simulink model "RS_O_yalmip"  (R2016b)
settings: Solver=ode1  StartTime=0.0  StopTime=T  FixedStep=1e-4  MaxStep=1e-3  RelTol=1e-6  EnableMultiTasking=on
InitFcn:
  | RS_O_script;
values from neighbouring files (symbols this model uses):
  C1 = 1e-9    (= 1e-09)    [Dati_MPC.m]
  C2 = 1e-9    (= 1e-09)    [Dati_MPC.m]
  Cext_Bp1 = Ce_Bp1*np_Bp1/ns_Bp1    (= 35750)    [Dati_MPC.m]
  Cext_Bp2 = Ce_Bp2*np_Bp2/ns_Bp2    (= 35750)    [Dati_MPC.m]
  Cext_BpM = Ce_BpM*np_BpM/ns_BpM    (= 68250)    [Dati_MPC.m]
  Cin_Bp1 = Ci_Bp1*np_Bp1/ns_Bp1    (= 16500)    [Dati_MPC.m]
  Cin_Bp2 = Ci_Bp2*np_Bp2/ns_Bp2    (= 16500)    [Dati_MPC.m]
  Cin_BpM = Ci_BpM*np_BpM/ns_BpM    (= 31500)    [Dati_MPC.m]
  Cint = 18e-3    (= 0.018)    [Dati_MPC.m]
  f = 50    [Dati_rete.m]
  ft_F = 10    [Dati_MPC.m]
  I_u = 0.1    [Dati_MPC.m]
  ki_PLL = w_t/Vd*(-w_t+sqrt(2*w_t^2-Vd^2*kp_PLL^2))    [Dati_MPC.m]
  kp_PLL = 0.9*kp_PLL_max    [Dati_MPC.m]
  MPCpar = struct    [Dati_MPC.m]    (also in Initialization.m)
  netdata = struct    [Dati_rete.m]
  P1 = 750e3    (= 750000)    [RS_O_script.m]
  P1v = 500e3    (= 500000)    [RS_O_script.m]
  P2 = 750e3    (= 750000)    [RS_O_script.m]
  P2v = 250e3    (= 250000)    [RS_O_script.m]
  P_u = 0.005    [Dati_MPC.m]
  Ppv1 = 500e3    (= 500000)    [Dati_MPC.m]
  Ppv2 = 850e3    (= 850000)    [Dati_MPC.m]
  Q1 = 350e3    (= 350000)    [RS_O_script.m]
  Q1v = 250e3    (= 250000)    [RS_O_script.m]
  Q2 = 300e3    (= 300000)    [RS_O_script.m]
  Q2v = 250e3    (= 250000)    [RS_O_script.m]
  Qbat1 = 50e3    (= 50000)    [Dati_MPC.m]
  Qbat2 = 50e3    (= 50000)    [Dati_MPC.m]
  Rext_Bp1 = Re_Bp1*ns_Bp1/np_Bp1    (= 0.0154545454545)    [Dati_MPC.m]
  Rext_Bp2 = Re_Bp2*ns_Bp2/np_Bp2    (= 0.0154545454545)    [Dati_MPC.m]
  Rext_BpM = Re_BpM*ns_BpM/np_BpM    (= 0.00809523809524)    [Dati_MPC.m]
  Rin_Bp1 = Ri_Bp1*ns_Bp1/np_Bp1    (= 0.363636363636)    [Dati_MPC.m]
  Rin_Bp2 = Ri_Bp2*ns_Bp2/np_Bp2    (= 0.363636363636)    [Dati_MPC.m]
  Rin_BpM = Ri_BpM*ns_BpM/np_BpM    (= 0.190476190476)    [Dati_MPC.m]
  SOC_10 = (Vbat1-Vbat1_min)/(Vbat1_max-Vbat1_min)    (= 0.625)    [Dati_MPC.m]
  SOC_20 = (Vbat2-Vbat2_min)/(Vbat2_max-Vbat2_min)    (= 0.625)    [Dati_MPC.m]
  SOC_M0 = (VbatM-VbatM_min)/(VbatM_max-VbatM_min)    (= 0.625)    [Dati_MPC.m]
  Srif = 1e6    (= 1000000)    [Dati_rete.m]
  t1 = 50    [RS_O_script.m]
  t2 = 110    [RS_O_script.m]
  t3 = 170    [RS_O_script.m]
  t_start_MPC = 10    [RS_O_script.m]
  tPLL = 2    [RS_O_script.m]
  Vbat1_max = 1.2*Vbat1_min    (= 480)    [Dati_MPC.m]
  Vbat1_min = 400    [Dati_MPC.m]
  Vbat2_max = 1.2*Vbat2_min    (= 480)    [Dati_MPC.m]
  Vbat2_min = 400    [Dati_MPC.m]
  VbatM_max = 1.2*VbatM_min    (= 480)    [Dati_MPC.m]
  VbatM_min = 400    [Dati_MPC.m]
  Vdc_1 = 800    [Dati_MPC.m]
  Vdc_2 = 800    [Dati_MPC.m]
  Vdc_M = 800    [Dati_MPC.m]
  Vrif_M = sqrt(2)/sqrt(3)*20e3    [Dati_MPC.m]
  Zrif = Vrif^2/Srif    (= 400)    [Dati_rete.m]
undefined symbols (not defined in the file or in its folder): Cfsc, Csc, j, L2, Lf, magnitude, Rc, Rint, Rsc
libraries: powerlib x87, powerlib_meascontrol x58, simulink x2
(part 3 of 3)

== system RS_O_yalmip/Misure 1/Filtro_c ==
  In : Inport
  Complex to Real-Imag : ComplexToRealImag
  First-Order Filter : powerlib_meascontrol/Filters/First-Order Filter  FilterType=Lowpass  Tc=1/(2*pi*ft_F)  Ts=0  Initialize=on  Vac_Init=[0, 0, 60]  Vdc_Init=0  PlotResponse=off  FreqRange="[0,  200,  1]"
  First-Order Filter1 : powerlib_meascontrol/Filters/First-Order Filter  FilterType=Lowpass  Tc=1/(2*pi*ft_F)  Ts=0  Initialize=on  Vac_Init=[0, 0, 60]  Vdc_Init=0  PlotResponse=off  FreqRange="[0,  200,  1]"
  Real-Imag to Complex : RealImagToComplex
  Out : Outport
  wires:
  Complex to Real-Imag/2 -> First-Order Filter1/1
  First-Order Filter/1 -> Real-Imag to Complex/1
  Complex to Real-Imag/1 -> First-Order Filter/1
  First-Order Filter1/1 -> Real-Imag to Complex/2
  Real-Imag to Complex/1 -> Out/1
  In/1 -> Complex to Real-Imag/1

== system RS_O_yalmip/Misure 1/Filtro_c1 ==
  In : Inport
  Complex to Real-Imag : ComplexToRealImag
  First-Order Filter : powerlib_meascontrol/Filters/First-Order Filter  FilterType=Lowpass  Tc=1/(2*pi*ft_F)  Ts=0  Initialize=on  Vac_Init=[0, 0, 60]  Vdc_Init=0  PlotResponse=off  FreqRange="[0,  200,  1]"
  First-Order Filter1 : powerlib_meascontrol/Filters/First-Order Filter  FilterType=Lowpass  Tc=1/(2*pi*ft_F)  Ts=0  Initialize=on  Vac_Init=[0, 0, 60]  Vdc_Init=0  PlotResponse=off  FreqRange="[0,  200,  1]"
  Real-Imag to Complex : RealImagToComplex
  Out : Outport
  wires:
  In/1 -> Complex to Real-Imag/1
  Real-Imag to Complex/1 -> Out/1
  First-Order Filter1/1 -> Real-Imag to Complex/2
  Complex to Real-Imag/1 -> First-Order Filter/1
  First-Order Filter/1 -> Real-Imag to Complex/1
  Complex to Real-Imag/2 -> First-Order Filter1/1

== system RS_O_yalmip/Misure 1/I Park assi sincroni1 ==
  I_1,2,3 : Inport
  Fase_rete : Inport  Port=2
  Add : Sum  Inputs=+++
  Constant : Constant  Value=exp(j*2*pi/3)
  Constant1 : Constant  Value=exp(j*4*pi/3)
  Demux : Demux  Outputs=3
  Gain : Gain  Gain=2/3
  Gain1 : Gain  Gain=-j
  Math Function : Math  SaturateOnIntegerOverflow=on
  Product : Product
  Product1 : Product
  Product2 : Product
  I_d,q : Outport
  wires:
  Math Function/1 -> Product2/2
  Fase_rete/1 -> Gain1/1
  Product2/1 -> I_d,q/1
  Gain1/1 -> Math Function/1
  Gain/1 -> Product2/1
  Product/1 -> Add/2
  Product1/1 -> Add/3
  Constant/1 -> Product/2
  Constant1/1 -> Product1/2
  Add/1 -> Gain/1
  I_1,2,3/1 -> Demux/1
  Demux/1 -> Add/1
  Demux/2 -> Product/1
  Demux/3 -> Product1/1

== system RS_O_yalmip/Misure 1/Subsystem1 ==
  V_dq : Inport
  I_dq : Inport  Port=2
  Divide2 : Product  Inputs=**
  Gain : Gain  Gain=3/2
  Math Function : Math  Operator=conj  SaturateOnIntegerOverflow=on
  P,Q : Outport
  wires:
  Divide2/1 -> Gain/1
  Gain/1 -> P,Q/1
  Math Function/1 -> Divide2/2
  V_dq/1 -> Divide2/1
  I_dq/1 -> Math Function/1

== system RS_O_yalmip/Misure 1/V Park assi sincroni ==
  V_c_1,2,3 : Inport
  Fase_rete : Inport  Port=2
  Add : Sum  Inputs=+++
  Constant : Constant  Value=exp(j*2*pi/3)
  Constant1 : Constant  Value=exp(j*4*pi/3)
  Demux : Demux  Outputs=3
  Gain : Gain  Gain=2/3
  Gain1 : Gain  Gain=-j
  Math Function : Math  SaturateOnIntegerOverflow=on
  Product : Product
  Product1 : Product
  Product2 : Product
  Vc_d,q : Outport
  wires:
  Gain/1 -> Product2/1
  Demux/3 -> Product1/1
  Demux/2 -> Product/1
  Demux/1 -> Add/1
  V_c_1,2,3/1 -> Demux/1
  Add/1 -> Gain/1
  Constant1/1 -> Product1/2
  Constant/1 -> Product/2
  Product1/1 -> Add/3
  Product/1 -> Add/2
  Math Function/1 -> Product2/2
  Gain1/1 -> Math Function/1
  Product2/1 -> Vc_d,q/1
  Fase_rete/1 -> Gain1/1

== system RS_O_yalmip/Misure 2/Filtro_c ==
  In : Inport
  Complex to Real-Imag : ComplexToRealImag
  First-Order Filter : powerlib_meascontrol/Filters/First-Order Filter  FilterType=Lowpass  Tc=1/(2*pi*ft_F)  Ts=0  Initialize=on  Vac_Init=[0, 0, 60]  Vdc_Init=0  PlotResponse=off  FreqRange="[0,  200,  1]"
  First-Order Filter1 : powerlib_meascontrol/Filters/First-Order Filter  FilterType=Lowpass  Tc=1/(2*pi*ft_F)  Ts=0  Initialize=on  Vac_Init=[0, 0, 60]  Vdc_Init=0  PlotResponse=off  FreqRange="[0,  200,  1]"
  Real-Imag to Complex : RealImagToComplex
  Out : Outport
  wires:
  Complex to Real-Imag/2 -> First-Order Filter1/1
  First-Order Filter/1 -> Real-Imag to Complex/1
  Complex to Real-Imag/1 -> First-Order Filter/1
  First-Order Filter1/1 -> Real-Imag to Complex/2
  Real-Imag to Complex/1 -> Out/1
  In/1 -> Complex to Real-Imag/1

== system RS_O_yalmip/Misure 2/Filtro_c1 ==
  In : Inport
  Complex to Real-Imag : ComplexToRealImag
  First-Order Filter : powerlib_meascontrol/Filters/First-Order Filter  FilterType=Lowpass  Tc=1/(2*pi*ft_F)  Ts=0  Initialize=on  Vac_Init=[0, 0, 60]  Vdc_Init=0  PlotResponse=off  FreqRange="[0,  200,  1]"
  First-Order Filter1 : powerlib_meascontrol/Filters/First-Order Filter  FilterType=Lowpass  Tc=1/(2*pi*ft_F)  Ts=0  Initialize=on  Vac_Init=[0, 0, 60]  Vdc_Init=0  PlotResponse=off  FreqRange="[0,  200,  1]"
  Real-Imag to Complex : RealImagToComplex
  Out : Outport
  wires:
  In/1 -> Complex to Real-Imag/1
  Real-Imag to Complex/1 -> Out/1
  First-Order Filter1/1 -> Real-Imag to Complex/2
  Complex to Real-Imag/1 -> First-Order Filter/1
  First-Order Filter/1 -> Real-Imag to Complex/1
  Complex to Real-Imag/2 -> First-Order Filter1/1

== system RS_O_yalmip/Misure 2/I Park assi sincroni1 ==
  I_1,2,3 : Inport
  Fase_rete : Inport  Port=2
  Add : Sum  Inputs=+++
  Constant : Constant  Value=exp(j*2*pi/3)
  Constant1 : Constant  Value=exp(j*4*pi/3)
  Demux : Demux  Outputs=3
  Gain : Gain  Gain=2/3
  Gain1 : Gain  Gain=-j
  Math Function : Math  SaturateOnIntegerOverflow=on
  Product : Product
  Product1 : Product
  Product2 : Product
  I_d,q : Outport
  wires:
  Demux/3 -> Product1/1
  Demux/2 -> Product/1
  Demux/1 -> Add/1
  I_1,2,3/1 -> Demux/1
  Add/1 -> Gain/1
  Constant1/1 -> Product1/2
  Constant/1 -> Product/2
  Product1/1 -> Add/3
  Product/1 -> Add/2
  Gain/1 -> Product2/1
  Gain1/1 -> Math Function/1
  Product2/1 -> I_d,q/1
  Fase_rete/1 -> Gain1/1
  Math Function/1 -> Product2/2

== system RS_O_yalmip/Misure 2/Subsystem1 ==
  V_dq : Inport
  I_dq : Inport  Port=2
  Divide2 : Product  Inputs=**
  Gain : Gain  Gain=3/2
  Math Function : Math  Operator=conj  SaturateOnIntegerOverflow=on
  P,Q : Outport
  wires:
  I_dq/1 -> Math Function/1
  V_dq/1 -> Divide2/1
  Math Function/1 -> Divide2/2
  Gain/1 -> P,Q/1
  Divide2/1 -> Gain/1

== system RS_O_yalmip/Misure 2/V Park assi sincroni ==
  V_c_1,2,3 : Inport
  Fase_rete : Inport  Port=2
  Add : Sum  Inputs=+++
  Constant : Constant  Value=exp(j*2*pi/3)
  Constant1 : Constant  Value=exp(j*4*pi/3)
  Demux : Demux  Outputs=3
  Gain : Gain  Gain=2/3
  Gain1 : Gain  Gain=-j
  Math Function : Math  SaturateOnIntegerOverflow=on
  Product : Product
  Product1 : Product
  Product2 : Product
  Vc_d,q : Outport
  wires:
  Fase_rete/1 -> Gain1/1
  Product2/1 -> Vc_d,q/1
  Gain1/1 -> Math Function/1
  Math Function/1 -> Product2/2
  Product/1 -> Add/2
  Product1/1 -> Add/3
  Constant/1 -> Product/2
  Constant1/1 -> Product1/2
  Add/1 -> Gain/1
  V_c_1,2,3/1 -> Demux/1
  Demux/1 -> Add/1
  Demux/2 -> Product/1
  Demux/3 -> Product1/1
  Gain/1 -> Product2/1

== system RS_O_yalmip/Misure Master/Filtro_c ==
  In : Inport
  Complex to Real-Imag : ComplexToRealImag
  First-Order Filter : powerlib_meascontrol/Filters/First-Order Filter  FilterType=Lowpass  Tc=1/(2*pi*ft_F)  Ts=0  Initialize=on  Vac_Init=[0, 0, 60]  Vdc_Init=0  PlotResponse=off  FreqRange="[0,  200,  1]"
  First-Order Filter1 : powerlib_meascontrol/Filters/First-Order Filter  FilterType=Lowpass  Tc=1/(2*pi*ft_F)  Ts=0  Initialize=on  Vac_Init=[0, 0, 60]  Vdc_Init=0  PlotResponse=off  FreqRange="[0,  200,  1]"
  Real-Imag to Complex : RealImagToComplex
  Out : Outport
  wires:
  Complex to Real-Imag/2 -> First-Order Filter1/1
  First-Order Filter/1 -> Real-Imag to Complex/1
  Complex to Real-Imag/1 -> First-Order Filter/1
  First-Order Filter1/1 -> Real-Imag to Complex/2
  Real-Imag to Complex/1 -> Out/1
  In/1 -> Complex to Real-Imag/1

== system RS_O_yalmip/Misure Master/Filtro_c1 ==
  In : Inport
  Complex to Real-Imag : ComplexToRealImag
  First-Order Filter : powerlib_meascontrol/Filters/First-Order Filter  FilterType=Lowpass  Tc=1/(2*pi*ft_F)  Ts=0  Initialize=on  Vac_Init=[0, 0, 60]  Vdc_Init=0  PlotResponse=off  FreqRange="[0,  200,  1]"
  First-Order Filter1 : powerlib_meascontrol/Filters/First-Order Filter  FilterType=Lowpass  Tc=1/(2*pi*ft_F)  Ts=0  Initialize=on  Vac_Init=[0, 0, 60]  Vdc_Init=0  PlotResponse=off  FreqRange="[0,  200,  1]"
  Real-Imag to Complex : RealImagToComplex
  Out : Outport
  wires:
  In/1 -> Complex to Real-Imag/1
  Real-Imag to Complex/1 -> Out/1
  First-Order Filter1/1 -> Real-Imag to Complex/2
  Complex to Real-Imag/1 -> First-Order Filter/1
  First-Order Filter/1 -> Real-Imag to Complex/1
  Complex to Real-Imag/2 -> First-Order Filter1/1

== system RS_O_yalmip/Misure Master/I Park assi sincroni1 ==
  I_1,2,3 : Inport
  Fase_rete : Inport  Port=2
  Add : Sum  Inputs=+++
  Constant : Constant  Value=exp(j*2*pi/3)
  Constant1 : Constant  Value=exp(j*4*pi/3)
  Demux : Demux  Outputs=3
  Gain : Gain  Gain=2/3
  Gain1 : Gain  Gain=-j
  Math Function : Math  SaturateOnIntegerOverflow=on
  Product : Product
  Product1 : Product
  Product2 : Product
  I_d,q : Outport
  I_ab : Outport  Port=2
  wires:
  Demux/3 -> Product1/1
  Demux/2 -> Product/1
  Demux/1 -> Add/1
  I_1,2,3/1 -> Demux/1
  Add/1 -> Gain/1
  Constant1/1 -> Product1/2
  Constant/1 -> Product/2
  Product1/1 -> Add/3
  Product/1 -> Add/2
  Gain/1 -> I_ab/1, Product2/1
  Gain1/1 -> Math Function/1
  Product2/1 -> I_d,q/1
  Fase_rete/1 -> Gain1/1
  Math Function/1 -> Product2/2

== system RS_O_yalmip/Misure Master/Subsystem1 ==
  V_dq : Inport
  I_dq : Inport  Port=2
  Divide2 : Product  Inputs=**
  Gain : Gain  Gain=3/2
  Math Function : Math  Operator=conj  SaturateOnIntegerOverflow=on
  P,Q : Outport
  wires:
  I_dq/1 -> Math Function/1
  V_dq/1 -> Divide2/1
  Math Function/1 -> Divide2/2
  Gain/1 -> P,Q/1
  Divide2/1 -> Gain/1

== system RS_O_yalmip/Misure Master/V Park assi sincroni ==
  V_c_1,2,3 : Inport
  Fase_rete : Inport  Port=2
  Add : Sum  Inputs=+++
  Constant : Constant  Value=exp(j*2*pi/3)
  Constant1 : Constant  Value=exp(j*4*pi/3)
  Demux : Demux  Outputs=3
  Gain : Gain  Gain=2/3
  Gain1 : Gain  Gain=-j
  Math Function : Math  SaturateOnIntegerOverflow=on
  Product : Product
  Product1 : Product
  Product2 : Product
  Vc_d,q : Outport
  wires:
  Fase_rete/1 -> Gain1/1
  Product2/1 -> Vc_d,q/1
  Gain1/1 -> Math Function/1
  Math Function/1 -> Product2/2
  Product/1 -> Add/2
  Product1/1 -> Add/3
  Constant/1 -> Product/2
  Constant1/1 -> Product1/2
  Add/1 -> Gain/1
  V_c_1,2,3/1 -> Demux/1
  Demux/1 -> Add/1
  Demux/2 -> Product/1
  Demux/3 -> Product1/1
  Gain/1 -> Product2/1

== system RS_O_yalmip/Misure transito/Subsystem2 ==
  V_c : Inport
  Add : Sum  Inputs=+-
  Add1 : Sum  Inputs=+-
  Add2 : Sum  Inputs=+-
  Demux : Demux  Outputs=3
  Gain : Gain  Gain=1/3
  Gain1 : Gain  Gain=1/3
  Gain2 : Gain  Gain=1/3
  Mux2 : Mux  Inputs=3
  V_f : Outport
  wires:
  Demux/3 -> Gain2/1
  V_c/1 -> Demux/1
  Add2/1 -> Mux2/3
  Add1/1 -> Mux2/2
  Add/1 -> Mux2/1
  Gain1/1 -> Add1/1, Add2/2
  Gain2/1 -> Add2/1, Add/2
  Demux/2 -> Gain1/1
  Gain/1 -> Add/1, Add1/2
  Demux/1 -> Gain/1
  Mux2/1 -> V_f/1

== system RS_O_yalmip/Carico1/PLL/Filtro_c ==
  In : Inport
  Complex to Real-Imag : ComplexToRealImag
  Real-Imag to Complex : RealImagToComplex
  Second-Order Filter{1..4} (4 alike) : powerlib_meascontrol/Filters/Second-Order Filter  FilterType=Lowpass  Fo=ft_PLL  Zeta=0.707  Ts=0  Initialize=on  Vac_Init="[0,  0,  60]"  Vdc_Init=Vrif_M  PlotResponse=off  FreqRange=[0, 500, 1]
  Out : Outport
  wires:
  Complex to Real-Imag/2 -> Second-Order Filter3/1
  Second-Order Filter3/1 -> Second-Order Filter4/1
  Second-Order Filter2/1 -> Real-Imag to Complex/1
  Second-Order Filter1/1 -> Second-Order Filter2/1
  Second-Order Filter4/1 -> Real-Imag to Complex/2
  Real-Imag to Complex/1 -> Out/1
  In/1 -> Complex to Real-Imag/1
  Complex to Real-Imag/1 -> Second-Order Filter1/1

== system RS_O_yalmip/Carico1/PLL/PI_fase ==
  dI : Inport
  Add1 : Sum
  Constant : Constant  Value=ki_PLL
  Constant1 : Constant  Value=kp_PLL
  Integrator : Integrator  LimitOutput=on  UpperSaturationLimit=30  LowerSaturationLimit=-30
  Product : Product
  Product1 : Product
  dw : Outport
  wires:
  Add1/1 -> dw/1
  dI/1 -> Product/2, Product1/1
  Integrator/1 -> Add1/2
  Product1/1 -> Integrator/1
  Constant/1 -> Product1/2
  Product/1 -> Add1/1
  Constant1/1 -> Product/1

== system RS_O_yalmip/Carico2/PLL/Filtro_c ==
  In : Inport
  Complex to Real-Imag : ComplexToRealImag
  Real-Imag to Complex : RealImagToComplex
  Second-Order Filter{1..4} (4 alike) : powerlib_meascontrol/Filters/Second-Order Filter  FilterType=Lowpass  Fo=ft_PLL  Zeta=0.707  Ts=0  Initialize=on  Vac_Init="[0,  0,  60]"  Vdc_Init=Vrif_M  PlotResponse=off  FreqRange=[0, 500, 1]
  Out : Outport
  wires:
  Complex to Real-Imag/2 -> Second-Order Filter3/1
  Second-Order Filter3/1 -> Second-Order Filter4/1
  Second-Order Filter2/1 -> Real-Imag to Complex/1
  Second-Order Filter1/1 -> Second-Order Filter2/1
  Second-Order Filter4/1 -> Real-Imag to Complex/2
  Real-Imag to Complex/1 -> Out/1
  In/1 -> Complex to Real-Imag/1
  Complex to Real-Imag/1 -> Second-Order Filter1/1

== system RS_O_yalmip/Carico2/PLL/PI_fase ==
  dI : Inport
  Add1 : Sum
  Constant : Constant  Value=ki_PLL
  Constant1 : Constant  Value=kp_PLL
  Integrator : Integrator  LimitOutput=on  UpperSaturationLimit=30  LowerSaturationLimit=-30
  Product : Product
  Product1 : Product
  dw : Outport
  wires:
  Add1/1 -> dw/1
  dI/1 -> Product/2, Product1/1
  Integrator/1 -> Add1/2
  Product1/1 -> Integrator/1
  Constant/1 -> Product1/2
  Product/1 -> Add1/1
  Constant1/1 -> Product/1

== system RS_O_yalmip/Controllo 1/PLL/Filtro_c ==
  In : Inport
  Complex to Real-Imag : ComplexToRealImag
  Real-Imag to Complex : RealImagToComplex
  Second-Order Filter{1..4} (4 alike) : powerlib_meascontrol/Filters/Second-Order Filter  FilterType=Lowpass  Fo=ft_PLL  Zeta=0.707  Ts=0  Initialize=on  Vac_Init="[0,  0,  60]"  Vdc_Init=Vrif_M  PlotResponse=off  FreqRange=[0, 500, 1]
  Out : Outport
  wires:
  Complex to Real-Imag/2 -> Second-Order Filter3/1
  Second-Order Filter3/1 -> Second-Order Filter4/1
  Second-Order Filter2/1 -> Real-Imag to Complex/1
  Second-Order Filter1/1 -> Second-Order Filter2/1
  Second-Order Filter4/1 -> Real-Imag to Complex/2
  Real-Imag to Complex/1 -> Out/1
  In/1 -> Complex to Real-Imag/1
  Complex to Real-Imag/1 -> Second-Order Filter1/1

== system RS_O_yalmip/Controllo 1/PLL/PI_fase ==
  dI : Inport
  Add1 : Sum
  Constant : Constant  Value=ki_PLL
  Constant1 : Constant  Value=kp_PLL
  Integrator : Integrator  LimitOutput=on  UpperSaturationLimit=30  LowerSaturationLimit=-30
  Product : Product
  Product1 : Product
  dw : Outport
  wires:
  Add1/1 -> dw/1
  dI/1 -> Product/2, Product1/1
  Integrator/1 -> Add1/2
  Product1/1 -> Integrator/1
  Constant/1 -> Product1/2
  Product/1 -> Add1/1
  Constant1/1 -> Product/1

== system RS_O_yalmip/Controllo 2/PLL/Filtro_c ==
  In : Inport
  Complex to Real-Imag : ComplexToRealImag
  Real-Imag to Complex : RealImagToComplex
  Second-Order Filter{1..4} (4 alike) : powerlib_meascontrol/Filters/Second-Order Filter  FilterType=Lowpass  Fo=ft_PLL  Zeta=0.707  Ts=0  Initialize=on  Vac_Init="[0,  0,  60]"  Vdc_Init=Vrif_M  PlotResponse=off  FreqRange=[0, 500, 1]
  Out : Outport
  wires:
  Complex to Real-Imag/2 -> Second-Order Filter3/1
  Second-Order Filter3/1 -> Second-Order Filter4/1
  Second-Order Filter2/1 -> Real-Imag to Complex/1
  Second-Order Filter1/1 -> Second-Order Filter2/1
  Second-Order Filter4/1 -> Real-Imag to Complex/2
  Real-Imag to Complex/1 -> Out/1
  In/1 -> Complex to Real-Imag/1
  Complex to Real-Imag/1 -> Second-Order Filter1/1

== system RS_O_yalmip/Controllo 2/PLL/PI_fase ==
  dI : Inport
  Add1 : Sum
  Constant : Constant  Value=ki_PLL
  Constant1 : Constant  Value=kp_PLL
  Integrator : Integrator  LimitOutput=on  UpperSaturationLimit=30  LowerSaturationLimit=-30
  Product : Product
  Product1 : Product
  dw : Outport
  wires:
  Add1/1 -> dw/1
  dI/1 -> Product/2, Product1/1
  Integrator/1 -> Add1/2
  Product1/1 -> Integrator/1
  Constant/1 -> Product1/2
  Product/1 -> Add1/1
  Constant1/1 -> Product/1

== system RS_O_yalmip/Controllo Master/Media complessa/Filtro_c1 ==
  In : Inport
  Complex to Real-Imag : ComplexToRealImag
  First-Order Filter : powerlib_meascontrol/Filters/First-Order Filter  FilterType=Lowpass  Tc=1/(2*pi*5)  Ts=0  Initialize=off  Vac_Init=[0, 0, 60]  Vdc_Init=0  PlotResponse=off  FreqRange="[0,  200,  1]"
  First-Order Filter1 : powerlib_meascontrol/Filters/First-Order Filter  FilterType=Lowpass  Tc=1/(2*pi*5)  Ts=0  Initialize=off  Vac_Init=[0, 0, 60]  Vdc_Init=0  PlotResponse=off  FreqRange="[0,  200,  1]"
  Real-Imag to Complex : RealImagToComplex
  Out : Outport
  wires:
  Complex to Real-Imag/2 -> First-Order Filter1/1
  Real-Imag to Complex/1 -> Out/1
  In/1 -> Complex to Real-Imag/1
  Complex to Real-Imag/1 -> First-Order Filter/1
  First-Order Filter/1 -> Real-Imag to Complex/1
  First-Order Filter1/1 -> Real-Imag to Complex/2
